simulink model "P2"  (R2022a)
settings: Solver=VariableStepAuto  StartTime=0.0  StopTime=10.0  RelTol=1e-3
libraries: spsSeriesRLCBranchLib x3, spsCurrentMeasurementLib x1, spsDCVoltageSourceLib x1, spsIGBTDiodeLib x1, simulink x1, spsVoltageMeasurementLib x1, spspowerguiLib x1
settings Model: Creator=Shiva  LastModifiedBy=Shiva

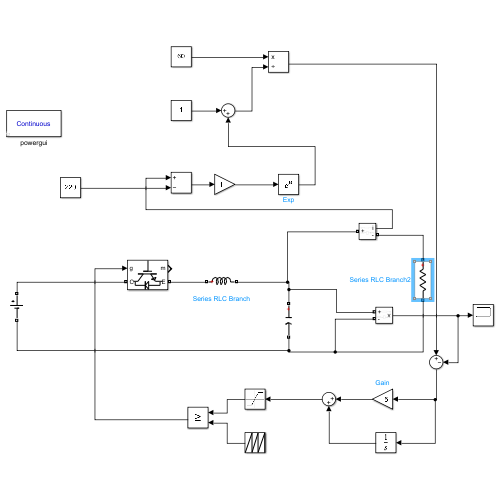
[thumbnail: Simulink's stored preview of the top-level diagram]
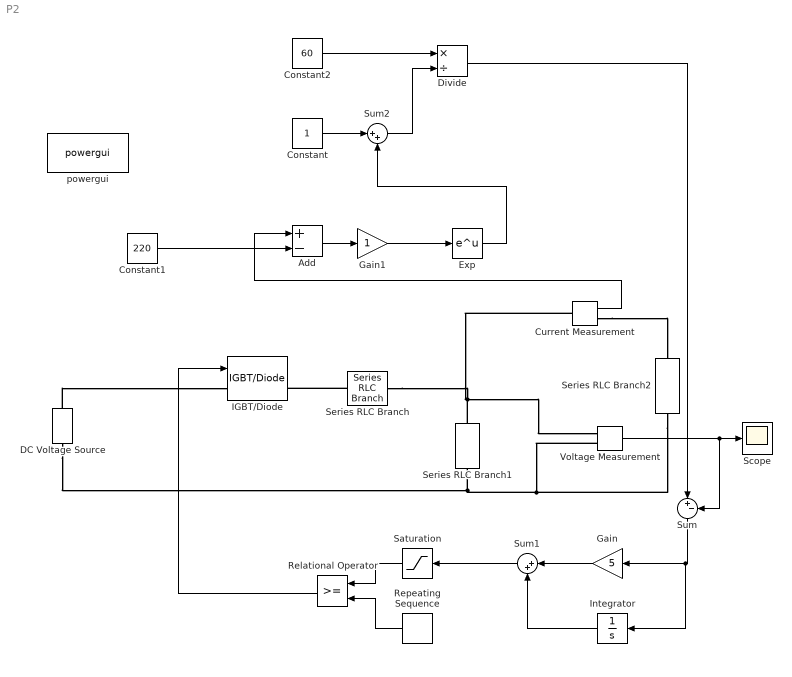
== system P2 ==
  Add : Sum  Inputs=+-
  Constant : Constant
  Constant1 : Constant  Value=220
  Constant2 : Constant  Value=60
  Current Measurement : spsCurrentMeasurementLib/Current Measurement  PhasorSimulation=off  OutputType=Complex  PSBequivalent=0
  DC Voltage Source : spsDCVoltageSourceLib/DC Voltage Source  Amplitude=120  Measurements=None
  Divide : Product  Inputs=*/
  Exp : Math
  Gain : Gain  Gain=5
  Gain1 : Gain
  IGBT/Diode : spsIGBTDiodeLib/IGBT//Diode  Ron=1e-3  Rs=1e5  Cs=inf  Measurements=on
  Integrator : Integrator
  Relational Operator : RelationalOperator  OutDataTypeStr=boolean  RndMeth=Simplest  InputSameDT=off
  Repeating Sequence : simulink/Sources/Repeating Sequence  rep_seq_t=[0 2]  rep_seq_y=[0 2]
  Saturation : Saturate
  Scope : Scope
  Series RLC Branch : spsSeriesRLCBranchLib/Series RLC Branch  LConnTagsString=__new0  RConnTagsString=__new0  BranchType=L  Resistance=1  Inductance=20e-3  SetiL0=off  InitialCurrent=0  Capacitance=1e-6  Setx0=off  InitialVoltage=0  Measurements=None
  Series RLC Branch1 : spsSeriesRLCBranchLib/Series RLC Branch  LConnTagsString=__new0  RConnTagsString=__new0  BranchType=C  Resistance=1  Inductance=1e-3  SetiL0=off  InitialCurrent=0  Capacitance=0.5  Setx0=off  InitialVoltage=0  Measurements=None
  Series RLC Branch2 : spsSeriesRLCBranchLib/Series RLC Branch  LConnTagsString=__new0  RConnTagsString=__new0  BranchType=R  Resistance=100  Inductance=1e-3  SetiL0=off  InitialCurrent=0  Capacitance=1e-6  Setx0=off  InitialVoltage=0  Measurements=None
  Sum : Sum  Inputs=|+-
  Sum1 : Sum  Inputs=|++
  Sum2 : Sum  Inputs=|++
  Voltage Measurement : spsVoltageMeasurementLib/Voltage Measurement  PhasorSimulation=off  OutputType=Complex  PSBequivalent=0
  powergui : spspowerguiLib/powergui  Priority=1  SimulationMode=Continuous  SampleTime=50e-6  frequency=60  Iterations=50  frequencyindice=0  Pbase=100e6  ErrMax=1e-4  UnitsV=kV  UnitsW=MW  buscounter=0  FunctionMessages=off  echomessages=off  EnableUseOfTLC=off  CurrentSourceSwitches=off  DisableSnubberDevices=off  DisableRonSwitches=off  DisableVfSwitches=off  DisplayEquations=off  AutomaticDiscreteSolvers=off  SolverType=Tustin/Backward Euler (TBE)  Interpol=off  ExternalGateDelay=off  methode=off  Ts=100  x0status=blocks  SPID=on  SwTol=0  HookPort=off  NonlinearTolerance=1e-4  nMaxIteration=100  ContinueOnMaxIteration=off  RestoreLinks=warning  ResistiveCurrentMeasurement=off  Frange=[0:2:500]  Ylog=off  Xlog=on  ShowGrid=off  save=off  variable=ZData  structure=0  ZoomFFT=off  StartTime=0.0  cycles=1  DisplayStyle=1  fundamental=60  FreqAxis=off  MaxFrequency=1000  frequencyindicesteady=1  RmsSteady=1  display=off
  wires:
  Saturation/1 -> Relational Operator/1
  Repeating Sequence/1 -> Relational Operator/2
  Sum1/1 -> Saturation/1
  Gain/1 -> Sum1/1
  Integrator/1 -> Sum1/2
  Sum/1 -> Integrator/1, Gain/1
  Voltage Measurement/1 -> Sum/2, Scope/1
  Divide/1 -> Sum/1
  Relational Operator/1 -> IGBT/Diode/1
  Current Measurement/1 -> Add/1
  Gain1/1 -> Exp/1
  Add/1 -> Gain1/1
  Constant/1 -> Sum2/1
  Exp/1 -> Sum2/2
  Sum2/1 -> Divide/2
  Constant1/1 -> Add/2
  Constant2/1 -> Divide/1
  connections:
  Series RLC Branch/LConn1 -- IGBT/Diode/RConn1
  Series RLC Branch1/LConn1 -- Current Measurement/LConn1 -- Series RLC Branch/RConn1 -- Voltage Measurement/LConn1
  Voltage Measurement/LConn2 -- DC Voltage Source/LConn1 -- Series RLC Branch1/RConn1 -- Series RLC Branch2/RConn1
  DC Voltage Source/RConn1 -- IGBT/Diode/LConn1
  Current Measurement/RConn1 -- Series RLC Branch2/LConn1
